simulink model "D53_LKAS_JLU_20200910_1510"  (R2018b)
settings: Solver=ode3  StartTime=0.0  StopTime=10.0  FixedStep=0.01  RelTol=1e-3  EnableMultiTasking=on
model workspace (MAT data in the model file):
  MCOS : class17 (value not decoded)
  MCOS : class17 (value not decoded)
  MCOS : class17 (value not decoded)
  MCOS : class17 (value not decoded)
  MCOS : class17 (value not decoded)
  MCOS : class17 (value not decoded)
  MCOS : class17 (value not decoded)
  MCOS : class17 (value not decoded)
  MCOS : class17 (value not decoded)
  MCOS : class17 (value not decoded)
  MCOS : class17 (value not decoded)
  MCOS : class17 (value not decoded)
  MCOS : class17 (value not decoded)
  MCOS : class17 (value not decoded)
  MCOS : class17 (value not decoded)
  MCOS : class17 (value not decoded)
  MCOS : class17 (value not decoded)
  MCOS : class17 (value not decoded)
  MCOS : class17 (value not decoded)
  MCOS : class17 (value not decoded)
  MCOS : class17 (value not decoded)
  MCOS : class17 (value not decoded)
  MCOS : class17 (value not decoded)
  MCOS : class17 (value not decoded)
  MCOS : class17 (value not decoded)
  MCOS : class17 (value not decoded)
  MCOS : class17 (value not decoded)
  MCOS : class17 (value not decoded)
  MCOS : class17 (value not decoded)
  MCOS : class17 (value not decoded)
  MCOS : class17 (value not decoded)
  MCOS : class17 (value not decoded)
  MCOS : class17 (value not decoded)
  MCOS : class17 (value not decoded)
  MCOS : class17 (value not decoded)
  MCOS : class17 (value not decoded)
  MCOS : class17 (value not decoded)
  MCOS : class17 (value not decoded)
  MCOS : class17 (value not decoded)
  MCOS : class17 (value not decoded)
  MCOS : class17 (value not decoded)
  MCOS : class17 (value not decoded)
  MCOS : class17 (value not decoded)
  MCOS : class17 (value not decoded)
  MCOS : class17 (value not decoded)
  MCOS : class17 (value not decoded)
  MCOS : class17 (value not decoded)
  MCOS : class17 (value not decoded)
  MCOS : class17 (value not decoded)
  MCOS : class17 (value not decoded)
  MCOS : class17 (value not decoded)
  MCOS : class17 (value not decoded)
  MCOS : class17 (value not decoded)
  MCOS : class17 (value not decoded)
  MCOS : class17 (value not decoded)
  MCOS : class17 (value not decoded)
  MCOS : class17 (value not decoded)
  MCOS : class17 (value not decoded)
  MCOS : class17 (value not decoded)
  MCOS : class17 (value not decoded)
  MCOS : class17 (value not decoded)
  MCOS : class17 (value not decoded)
  MCOS : class17 (value not decoded)
  MCOS : class17 (value not decoded)
  MCOS : class17 (value not decoded)
  MCOS : class17 (value not decoded)
  MCOS : class17 (value not decoded)
  MCOS : class17 (value not decoded)
  MCOS : class17 (value not decoded)
  MCOS : class17 (value not decoded)
  MCOS : class17 (value not decoded)
  MCOS : class17 (value not decoded)
  MCOS : class17 (value not decoded)
  MCOS : class17 (value not decoded)
  MCOS : class17 (value not decoded)
  MCOS : class17 (value not decoded)
  MCOS : class17 (value not decoded)
  MCOS : class17 (value not decoded)
  MCOS : class17 (value not decoded)
  MCOS : class17 (value not decoded)
  MCOS : class17 (value not decoded)
  MCOS : class17 (value not decoded)
  MCOS : class17 (value not decoded)
  MCOS : class17 (value not decoded)
  MCOS : class17 (value not decoded)
  MCOS : class17 (value not decoded)
  MCOS : class17 (value not decoded)
  MCOS : class17 (value not decoded)
  MCOS : class17 (value not decoded)
undefined symbols (not defined in the file): LKA_CarWidth, LKA_SampleTime, LKA_StrRatio_C, LKA_Veh2CamL_C, LKA_Veh2CamW_C, LKA_WhlBaseL_C, LL_CompSWA_C, LL_CrvtPrvwT_C, LL_DesDvt_C, LL_DvtComp_C, LL_DvtPrvwT_C, LL_DvtSpdDet_vDvtSpdMin_C, LL_HdAgExT_C, LL_HdAgPrvwT_C, LL_LAccMax_C, LL_LAccRMax_C, LL_LDW_EarliestWarnLine_C, LL_LDW_LatestWarnLine_C, LL_LDWS_SUPPRESS_HEADING, LL_LFClb_TFC_DiffCtlBalance, LL_LFClb_TFC_DiffCtrlMaxSWA, LL_LFClb_TFC_DiffCtrlRatio, LL_LFClb_TFC_facmGainLutGain1_C, LL_LFClb_TFC_facmGainLutGain2_C, LL_LFClb_TFC_facmIntegRatio, LL_LFClb_TFC_facmKlat_C, LL_LFClb_TFC_FfCtlRatio_C, LL_LFClb_TFC_phiIntegCtlMaxSWA_C, LL_LFClb_TFC_tiKlatPrvwT_C, LL_LFClb_TFC_vGainLutVehSpdLwr_C, LL_LFClb_TFC_vGainLutVehSpdUpr_C, LL_LKA_EarliestWarnLine_C, LL_LKA_LatestWarnLine_C, LL_LKAExPrcs_ExitC0Dvt, LL_LKAExPrcs_ExitC0Swt, LL_LKAExPrcs_tiExitTime1, LL_LKAExPrcs_tiExitTime2, LL_LKAExPrcs_tiExitTime3, LL_LKAS_OUT_OF_CONTROL_LAT_VEL, LL_LKAS_OUT_OF_CONTROL_TTLC, LL_LKASWASyn_M0, LL_LKASWASyn_M1, LL_LKASWASyn_M2, LL_LKASWASyn_M3K, LL_LKASWASyn_SWAaddMax, LL_LKASWASyn_T2, LL_LKASWASyn_tiTrqSwaRtTime, LL_LKASWASyn_tiTrqSwaTime, LL_LKASWASyn_TrqMax, LL_LKASWASyn_TrqSwaAddSwt, LL_LKASWASyn_TrqSwaRateDiff, LL_LSpdCompT_C, LL_lStpLngth_C, LL_MAX_DELAY_EPSSTAR_TIME, LL_MAX_DRIVER_TORQUE_DISABLE, LL_MAX_DRIVER_TORQUE_ENABLE, LL_MAX_LANE_WIDTH_DISABLE, LL_MAX_LANE_WIDTH_ENABLE, LL_MAX_LAT_ACC_DISABLE, LL_MAX_LAT_ACC_ENABLE ... (+30)
libraries: simulink x134, canmsglib x52, dspstat3 x3, simulink_extras x1
(part 13 of 18)

== system D53_LKAS_JLU_20200910_1510/LL/LLOn/LL State Determination (LLStateDet)/LL State Machine Conditions (LLSMCon)/Deactivation Condition (DeactvC)/Deactivation Condition Synthesis (DeactvCSyn) ==
  DeactvCSyn_stDACMode : Inport
  DeactvCSyn_stDvtThresActvFlgLDW : Inport  Port=2
  DeactvCSyn_stDvtThresActvFlgLKA : Inport  Port=3
  DvrTkCon_stDvrTkConFlg : Inport  Port=4
  DeactvCSyn_stEPSCFlg : Inport  Port=5
  DeactvCSyn_stExitFlg : Inport  Port=6
  Cast To Single : DataTypeConversion  OutDataTypeStr=uint8
  Cast To Single1 : DataTypeConversion  OutDataTypeStr=uint8
  Default Flag (DflFlg) : Subsystem  TreatAsAtomicUnit=on
  Default Flag (DflFlg)1 : Subsystem  TreatAsAtomicUnit=on
  If : If  NumInputs=2  IfExpression=(u1 ==1|u1==2)& u2 == 0
  If1 : If  NumInputs=4  IfExpression=u1 == 2 & (u3 == 1 | u4 == 1)
  LDW Deactivation Flag (LDWDeactvFlg) : Subsystem  TreatAsAtomicUnit=on
  LKA Deactivation Flag (LKADeactvFlg) : Subsystem  TreatAsAtomicUnit=on
  Logical Operator : Logic  Operator=OR  AllPortsSameDT=off  OutDataTypeStr=boolean
  Merge : Merge
  Merge1 : Merge
  DeactvCSyn_stLDWDeactvCSyn : Outport
  DeactvCSyn_stLKADeactvCSyn : Outport  Port=2
  wires:
  DeactvCSyn_stDvtThresActvFlgLDW/1 -> If/2
  Logical Operator/1 -> Cast To Single/1
  DvrTkCon_stDvrTkConFlg/1 -> Logical Operator/1
  Cast To Single/1 -> If1/3
  If1/1 -> LKA Deactivation Flag (LKADeactvFlg)/Action
  Default Flag (DflFlg)1/1(Out) -> Merge1/2
  LKA Deactivation Flag (LKADeactvFlg)/1(Out) -> Merge1/1
  DeactvCSyn_stExitFlg/1 -> Cast To Single1/1
  DeactvCSyn_stEPSCFlg/1 -> Logical Operator/2
  Merge1/1 -> DeactvCSyn_stLKADeactvCSyn/1
  If1/2 -> Default Flag (DflFlg)1/Action
  Default Flag (DflFlg)/1(Out) -> Merge/2
  Merge/1 -> DeactvCSyn_stLDWDeactvCSyn/1
  DeactvCSyn_stDvtThresActvFlgLKA/1 -> If1/2
  DeactvCSyn_stDACMode/1 -> If/1, If1/1
  If/2 -> Default Flag (DflFlg)/Action
  If/1 -> LDW Deactivation Flag (LDWDeactvFlg)/Action
  LDW Deactivation Flag (LDWDeactvFlg)/1(Out) -> Merge/1
  Cast To Single1/1 -> If1/4

== system D53_LKAS_JLU_20200910_1510/LL/LLOn/LL State Determination (LLStateDet)/LL State Machine Conditions (LLSMCon)/Deactivation Condition (DeactvC)/Deviation Threshold Condition (DvtThresCon) ==
  DvtThresCon_vVehSpd : Inport
  DvtThresCon_bsL0Info : Inport  Port=2
  DvtThresCon_bsR0Info : Inport  Port=3
  DvtThresCon_bsTTLCInfo : Inport  Port=4
  DvtThresCon_bsHdAgInfo : Inport  Port=5
  DvtThresCon_bsDvtThresClb : Inport  Port=6
  Active Lane Calculation (ActLanCalc) : Subsystem
  Bus Selector : BusSelector  OutputSignals=LftTTLC,RgtTTLC
  Bus Selector1 : BusSelector  OutputSignals=ActvCClb
  Bus Selector2 : BusSelector  OutputSignals=phiHdAgLft,phiHdAgRgt
  Deviation Calculation (DvtCalc) : Subsystem
  Deviation Speed Calculation (DvtSpdCalc) : Subsystem
  Deviation Threshold Judgement LDW (DvtThresJdg) : Subsystem
  Deviation Threshold Judgement LKA (DvtThresJdg) : Subsystem
  Saturation1 : Saturate  UpperLimit=1  LowerLimit=-1
  Saturation5 : Saturate  UpperLimit=1  LowerLimit=-1
  DvtThresCon_stDvtThresActvFlgLDW : Outport
  DvtThresCon_stDvtThresActvFlgLKA : Outport  Port=2
  wires:
  Saturation1/1 -> Deviation Threshold Judgement LDW (DvtThresJdg)/2(DvtThresJdg_lRgtDvt), Deviation Threshold Judgement LKA (DvtThresJdg)/2(DvtThresJdg_lRgtDvt)
  Bus Selector/1 -> Deviation Threshold Judgement LDW (DvtThresJdg)/5(DvtThresJdg_tiLftTTLC), Deviation Threshold Judgement LKA (DvtThresJdg)/5(DvtThresJdg_tiLftTTLC)  "<LftTTLC>"
  Saturation5/1 -> Deviation Threshold Judgement LDW (DvtThresJdg)/1(DvtThresJdg_lLftDvt), Deviation Threshold Judgement LKA (DvtThresJdg)/1(DvtThresJdg_lLftDvt)
  Deviation Speed Calculation (DvtSpdCalc)/2(DvtSpdCalc_vRgtDvtSpd) -> Deviation Threshold Judgement LDW (DvtThresJdg)/4(DvtThresJdg_vRgtDvtSpd), Deviation Threshold Judgement LKA (DvtThresJdg)/4(DvtThresJdg_vRgtDvtSpd)  "DvtSpdCalc_vRgtDvtSpd"
  Bus Selector/2 -> Deviation Threshold Judgement LDW (DvtThresJdg)/6(DvtThresJdg_tiRgtTTLC), Deviation Threshold Judgement LKA (DvtThresJdg)/6(DvtThresJdg_tiRgtTTLC)  "<RgtTTLC>"
  Deviation Speed Calculation (DvtSpdCalc)/1(DvtSpdCalc_vLftDvtSpd) -> Deviation Threshold Judgement LDW (DvtThresJdg)/3(DvtThresJdg_vLftDvtSpd), Deviation Threshold Judgement LKA (DvtThresJdg)/3(DvtThresJdg_vLftDvtSpd)  "DvtSpdCalc_vLftDvtSpd"
  Active Lane Calculation (ActLanCalc)/1(ActLanCalc_ActvCClbOut) -> Deviation Threshold Judgement LDW (DvtThresJdg)/7(DvtThresJdg_bsDvtThresClb), Deviation Threshold Judgement LKA (DvtThresJdg)/7(DvtThresJdg_bsDvtThresClb)
  Deviation Threshold Judgement LDW (DvtThresJdg)/1(DvtThresJdg_stDvtThresActvFlg) -> DvtThresCon_stDvtThresActvFlgLDW/1  "DvtThresActvFlg"
  Bus Selector2/2 -> Deviation Speed Calculation (DvtSpdCalc)/2(DvtSpdCalc_phiPrvwHdAgRgt)  "<phiHdAgRgt>"
  Bus Selector2/1 -> Deviation Speed Calculation (DvtSpdCalc)/1(DvtSpdCalc_phiPrvwHdAgLft)  "<phiHdAgLft>"
  DvtThresCon_bsHdAgInfo/1 -> Bus Selector2/1
  DvtThresCon_bsTTLCInfo/1 -> Bus Selector/1  "TTLCInfo"
  DvtThresCon_vVehSpd/1 -> Deviation Speed Calculation (DvtSpdCalc)/3(DvtSpdCalc_vVehSpd)
  DvtThresCon_bsDvtThresClb/1 -> Bus Selector1/1
  Deviation Threshold Judgement LKA (DvtThresJdg)/1(DvtThresJdg_stDvtThresActvFlg) -> DvtThresCon_stDvtThresActvFlgLKA/1  "DvtThresActvFlg"
  Deviation Calculation (DvtCalc)/2(DvtCalc_lRgtDvt) -> Saturation1/1  "DvtCalc_lRgtDvt"
  Deviation Calculation (DvtCalc)/1(DvtCalc_lLftDvt) -> Saturation5/1  "DvtCalc_lLftDvt"
  DvtThresCon_bsR0Info/1 -> Active Lane Calculation (ActLanCalc)/2(ActLanCalc_bsR0Info), Deviation Calculation (DvtCalc)/2(DvtCalc_bsR0Info)
  DvtThresCon_bsL0Info/1 -> Active Lane Calculation (ActLanCalc)/1(ActLanCalc_bsL0Info), Deviation Calculation (DvtCalc)/1(DvtCalc_bsL0Info)
  Bus Selector1/1 -> Active Lane Calculation (ActLanCalc)/3(ActLanCalc_ActvCClb)  "<ActvCClb>"

== system D53_LKAS_JLU_20200910_1510/LL/LLOn/LL State Determination (LLStateDet)/LL State Machine Conditions (LLSMCon)/Deactivation Condition (DeactvC)/Driver Take Condition (DvrTkCon) ==
  DvrTkCon_crPrvwCrvt : Inport
  DvrTkCon_stActvFlg : Inport  Port=2
  DvrTkCon_bsLLSMConClb : Inport  Port=3
  DvrTkCon_vVehSpd : Inport  Port=4
  DvrTkCon_bsEPSInfo : Inport  Port=5
  Abs1 : Abs
  Add : Sum
  Bus Selector1 : BusSelector  OutputSignals=EPS_SW_Trq
  Bus Selector2 : BusSelector  OutputSignals=DisblCClb.LL_MAX_DRIVER_TORQUE_DISABLE
  Bus Selector3 : BusSelector  OutputSignals=LKA_SampleTime
  Cast To Single : DataTypeConversion  OutDataTypeStr=uint16
  Cast To Single1 : DataTypeConversion  OutDataTypeStr=uint16
  Cast To Single2 : DataTypeConversion  LockScale=on
  Compare To Constant : simulink/Logic and Bit Operations/Compare To Constant  relop=>  const=0  OutDataTypeStr=boolean
  Constant : Constant  Value=0.005  OutDataTypeStr=single
  Constant1 : Constant  OutDataTypeStr=single
  Constant2 : Constant  Value=0.2  OutDataTypeStr=single
  Count : Subsystem
  Count 0.2s : Subsystem
  Divide : Product  Inputs=*/
  Divide1 : Product  Inputs=*/
  Divide2 : Product  Inputs=*/  OutDataTypeStr=single
  Logical Operator : Logic  AllPortsSameDT=off  OutDataTypeStr=boolean
  MATLAB Function : MATLAB Function  TreatAsAtomicUnit=on
  Memory : Memory  InheritSampleTime=on
  Saturation : Saturate  UpperLimit=0.005  LowerLimit=-0.005
  Time Delay (TDel) : Subsystem
  DvrTkCon_stDvrTkConFlg : Outport
  wires:
  Count/1(Out) -> Add/2
  Cast To Single1/1 -> Add/1
  Memory/1 -> Logical Operator/2
  Logical Operator/1 -> Count/Enable
  Compare To Constant/1 -> Count/1(Input), Logical Operator/1
  Add/1 -> Time Delay (TDel)/2(TDel_tiTDel)
  Cast To Single/1 -> Count 0.2s/2(Input1)
  Bus Selector2/1 -> MATLAB Function/4(DisableTrq)  "<LL_MAX_DRIVER_TORQUE_DISABLE>"
  Saturation/1 -> Abs1/1
  DvrTkCon_crPrvwCrvt/1 -> Saturation/1
  Divide2/1 -> Cast To Single2/1
  Constant/1 -> Divide2/2
  Cast To Single2/1 -> MATLAB Function/5(CrvtTrq)
  Abs1/1 -> Divide2/1
  Divide1/1 -> Cast To Single1/1
  Constant1/1 -> Divide1/1
  Constant2/1 -> Divide/1
  Bus Selector3/1 -> Divide/2, Divide1/2  "<LKA_SampleTime>"
  Divide/1 -> Cast To Single/1
  [LLClb_bsConstantClb] -> Bus Selector3/1
  Time Delay (TDel)/1(TDel_stFlgOut) -> Memory/1, DvrTkCon_stDvrTkConFlg/1
  Count 0.2s/1(Out) -> Time Delay (TDel)/1(TDel_stFlgIn)
  MATLAB Function/1(stDvrTkConFlg) -> Count 0.2s/1(Input), Count 0.2s/Enable
  DvrTkCon_bsLLSMConClb/1 -> Bus Selector2/1
  DvrTkCon_vVehSpd/1 -> MATLAB Function/3(VehSpd)
  Bus Selector1/1 -> MATLAB Function/2(EPSTrq)  "<EPS_SW_Trq>"
  DvrTkCon_stActvFlg/1 -> MATLAB Function/1(stActvFlg), Compare To Constant/1
  DvrTkCon_bsEPSInfo/1 -> Bus Selector1/1

== system D53_LKAS_JLU_20200910_1510/LL/LLOn/LL State Determination (LLStateDet)/LL State Machine Conditions (LLSMCon)/Deactivation Condition (DeactvC)/EPS Condition (EPSC) ==
  EPSC_bsLLSMConClb : Inport
  EPSC_bsEPSInfo : Inport  Port=2
  EPSC_bsLLState : Inport  Port=3
  Bus Selector : BusSelector  OutputSignals=EPS_LKA_State
  Bus Selector1 : BusSelector  OutputSignals=LKA_State
  Bus Selector2 : BusSelector  OutputSignals=DisblCClb.LL_TkOvStChk_tiTDelTime
  Bus Selector3 : BusSelector  OutputSignals=LKA_SampleTime
  Cast To Single1 : DataTypeConversion  OutDataTypeStr=uint16
  Compare To Constant : simulink/Logic and Bit Operations/Compare To Constant  relop=~=  const=3  OutDataTypeStr=boolean
  Compare To Constant1 : simulink/Logic and Bit Operations/Compare To Constant  relop===  const=4  OutDataTypeStr=boolean
  Compare To Constant2 : simulink/Logic and Bit Operations/Compare To Constant  relop===  const=5  OutDataTypeStr=boolean
  Divide : Product  Inputs=*/  OutDataTypeStr=single
  Logical Operator : Logic  Operator=OR  AllPortsSameDT=off  OutDataTypeStr=boolean
  Logical Operator1 : Logic  AllPortsSameDT=off  OutDataTypeStr=boolean
  Sum Condition1 : Subsystem  TreatAsAtomicUnit=on
  EPSC_stEPSCFlg : Outport
  wires:
  Cast To Single1/1 -> Sum Condition1/2(Sum)
  EPSC_bsLLSMConClb/1 -> Bus Selector2/1
  Divide/1 -> Cast To Single1/1
  [LLClb_bsConstantClb] -> Bus Selector3/1
  Bus Selector2/1 -> Divide/1  "<LL_TkOvStChk_tiTDelTime>"
  Bus Selector3/1 -> Divide/2  "<LKA_SampleTime>"
  Sum Condition1/1(Out) -> Logical Operator1/2
  Logical Operator/1 -> Sum Condition1/Enable, Sum Condition1/1(In)
  Compare To Constant/1 -> Logical Operator1/1
  Compare To Constant2/1 -> Logical Operator/2
  Compare To Constant1/1 -> Logical Operator/1
  Bus Selector1/1 -> Compare To Constant2/1, Compare To Constant1/1  "<LKA_State>"
  Bus Selector/1 -> Compare To Constant/1  "<EPS_LKA_State>"
  EPSC_bsLLState/1 -> Bus Selector1/1
  Logical Operator1/1 -> EPSC_stEPSCFlg/1
  EPSC_bsEPSInfo/1 -> Bus Selector/1

== system D53_LKAS_JLU_20200910_1510/LL/LLOn/LL State Determination (LLStateDet)/LL State Machine Conditions (LLSMCon)/Disable Condition (DisblC)/Disable Condition Synthesis (DisblCSyn) ==
  DisblCSyn_stDACMode : Inport
  DisblCSyn_stVehStateC : Inport  Port=2
  DisblCSyn_stLaneC : Inport  Port=3
  DisblCSyn_stDrvInttC : Inport  Port=4
  DisblCSyn_stLDWOwnC : Inport  Port=5
  DisblCSyn_stLKAOwnC : Inport  Port=6
  DisblCSyn_stLDWAlrmTOut : Inport  Port=7
  Cast To Single : DataTypeConversion  OutDataTypeStr=uint8
  Cast To Single1 : DataTypeConversion  OutDataTypeStr=uint8
  Cast To Single2 : DataTypeConversion  OutDataTypeStr=uint8
  If Action Subsystem1 : Subsystem  TreatAsAtomicUnit=on
  If Action Subsystem2 : Subsystem  TreatAsAtomicUnit=on
  If Action Subsystem3 : Subsystem  TreatAsAtomicUnit=on
  If Action Subsystem4 : Subsystem  TreatAsAtomicUnit=on
  If1 : If  NumInputs=2  IfExpression=(u1 ==1|u1==2)& u2 == 1
  If2 : If  NumInputs=2  IfExpression=u1 == 2 & u2 == 1
  Logical Operator1 : Logic  Operator=OR  AllPortsSameDT=off  OutDataTypeStr=boolean
  Logical Operator2 : Logic  Operator=OR  Inputs=3  AllPortsSameDT=off  OutDataTypeStr=boolean
  Logical Operator3 : Logic  Operator=OR  Inputs=3  AllPortsSameDT=off  OutDataTypeStr=boolean
  Merge1 : Merge
  Merge2 : Merge
  DisblCSyn_stLDWDisblCSyn : Outport
  DisblCSyn_stLKADisblCSyn : Outport  Port=2
  wires:
  Cast To Single2/1 -> If2/2
  Cast To Single1/1 -> If1/2
  Cast To Single/1 -> If1/1, If2/1
  DisblCSyn_stLDWAlrmTOut/1 -> Logical Operator3/2
  Merge2/1 -> DisblCSyn_stLKADisblCSyn/1
  Logical Operator1/1 -> Cast To Single2/1
  If Action Subsystem3/1(Out) -> Merge2/2
  If2/2 -> If Action Subsystem3/Action
  If2/1 -> If Action Subsystem1/Action
  If Action Subsystem1/1(Out) -> Merge2/1
  DisblCSyn_stLKAOwnC/1 -> Logical Operator1/2
  If Action Subsystem4/1(Out) -> Merge1/2
  Merge1/1 -> DisblCSyn_stLDWDisblCSyn/1
  If1/2 -> If Action Subsystem4/Action
  If1/1 -> If Action Subsystem2/Action
  If Action Subsystem2/1(Out) -> Merge1/1
  Logical Operator2/1 -> Logical Operator1/1, Logical Operator3/3
  DisblCSyn_stDACMode/1 -> Cast To Single/1
  Logical Operator3/1 -> Cast To Single1/1
  DisblCSyn_stLDWOwnC/1 -> Logical Operator3/1
  DisblCSyn_stDrvInttC/1 -> Logical Operator2/3
  DisblCSyn_stLaneC/1 -> Logical Operator2/2
  DisblCSyn_stVehStateC/1 -> Logical Operator2/1

== system D53_LKAS_JLU_20200910_1510/LL/LLOn/LL State Determination (LLStateDet)/LL State Machine Conditions (LLSMCon)/Disable Condition (DisblC)/Driver Intent Condition (DrvInttC) ==
  DrvInttC_bsInInfoSyn : Inport
  DrvInttC_bsLLSMConClb : Inport  Port=2
  DrvInttC_crPrvwCrvt : Inport  Port=3
  Bus Creator : BusCreator  Inputs=3
  Bus Selector : BusSelector  OutputSignals=bsSWAInfo.SW_Angle,bsVehMovInfo.ESC_LatAcc,bsVehMovInfo.ESC_LonAcc,bsEPSInfo,bsVehMovInfo.ESC_VehSpd
  Bus Selector1 : BusSelector  OutputSignals=DisblCClb.LL_MAX_STEER_ANGLE_DISABLE,DisblCClb.LL_MAX_STEER_SPEED_DISABLE,DisblCClb.LL_MAX_DRIVER_TORQUE_DISABLE,DisblCClb.LL_MAX_LAT_ACC_DISABLE,DisblCClb.LL_MAX_LONG_ACC_DISABLE,DisblCClb.LL_MAX_LONG_DECEL_DISABLE,DisblCClb.LL_TkOvStChk_tiTrqChkT,DisblCClb.LL_TkOvStChk_tiTDelTime
  Driver Action Condition Synthesis (DrvActnCSyn) : Subsystem  Description=|
      | Block Name: Driver Action Condition Synthesis
      | Ab.: DrvActnCSyn
      | No.: 1.1.1.3.3.5
      | Rev: 0.0.1
      | Update Date: 19-3-26
  Driver Action Detection (DrvActnDet) : Subsystem  Description=|
      | Block Name: Driver Action Detection
      | Ab.: DrvActnDet
      | No.: 1.1.1.3.3.1
      | Rev: 0.0.1
      | Update Date: 19-3-26
  Driver Release Detection (DrvRlsDet) : Subsystem  Description=|
      | Block Name: Driver Release Detection
      | Ab.: DrvRlsDet
      | No.: 1.1.1.2.3.2
      | Rev: 0.0.1
      | Update Date: 19-3-26
  Take-Over Steering Check (TkOvStChk) : Subsystem  Description=|
      | Block Name: Take-Over Steering Check
      | Ab.: TkOvStChk
      | No.: 1.1.1.3.3.4
      | Rev: 0.0.1
      | Update Date: 19-3-26
  DrvInttC_stDrvInttCSyn : Outport
  DrvInttCSyn : Outport  Port=2
  wires:
  Bus Creator/1 -> DrvInttCSyn/1
  Driver Action Detection (DrvActnDet)/2(DrvActnDet) -> Bus Creator/1  "DrvActnDet"
  Driver Release Detection (DrvRlsDet)/1(DrvRlsDet_stDrvRlsDetFlg) -> Driver Action Condition Synthesis (DrvActnCSyn)/2(DrvActnCSyn_stDrvRlsDetFlg), Bus Creator/2  "DRIVER_RELEASE"
  Take-Over Steering Check (TkOvStChk)/1(TkOvStChk_stTkOvStChk) -> Driver Action Condition Synthesis (DrvActnCSyn)/3(DrvActnCSyn_stTkOvStChk), Bus Creator/3  "TkOvStChk"
  DrvInttC_crPrvwCrvt/1 -> Take-Over Steering Check (TkOvStChk)/6(TkOvStChk_crPrvwCrvt)
  DrvInttC_bsInInfoSyn/1 -> Bus Selector/1
  Bus Selector/5 -> Take-Over Steering Check (TkOvStChk)/1(TkOvStChk_bsVehSpd)  "<ESC_VehSpd>"
  Bus Selector1/8 -> Take-Over Steering Check (TkOvStChk)/5(TkOvStChk_tiTDel_C)  "<LL_TkOvStChk_tiTDelTime>"
  Bus Selector1/7 -> Take-Over Steering Check (TkOvStChk)/4(TkOvStChk_tiTrqChkT_C)  "<LL_TkOvStChk_tiTrqChkT>"
  Bus Selector1/3 -> Take-Over Steering Check (TkOvStChk)/3(TkOvStChk_trqSWTrqMax_C)  "<LL_MAX_DRIVER_TORQUE_DISABLE>"
  Bus Selector/4 -> Driver Action Detection (DrvActnDet)/9(DrvActnDet_bsEPSInfo), Driver Release Detection (DrvRlsDet)/1(DrvRlsDet_bsEPSInfo), Take-Over Steering Check (TkOvStChk)/2(TkOvStChk_bsEPSInfo)  "<bsEPSInfo>"
  Bus Selector1/6 -> Driver Action Detection (DrvActnDet)/8(DrvActnDet_aFAccMin_C)  "<LL_MAX_LONG_DECEL_DISABLE>"
  Bus Selector1/5 -> Driver Action Detection (DrvActnDet)/7(DrvActnDet_aFAccMax_C)  "<LL_MAX_LONG_ACC_DISABLE>"
  Bus Selector1/4 -> Driver Action Detection (DrvActnDet)/6(DrvActnDet_aLAccMax_C)  "<LL_MAX_LAT_ACC_DISABLE>"
  Bus Selector1/2 -> Driver Action Detection (DrvActnDet)/5(DrvActnDet_dphiSWARateMax_C)  "<LL_MAX_STEER_SPEED_DISABLE>"
  Bus Selector1/1 -> Driver Action Detection (DrvActnDet)/4(DrvActnDet_phiSWAMax_C)  "<LL_MAX_STEER_ANGLE_DISABLE>"
  DrvInttC_bsLLSMConClb/1 -> Bus Selector1/1
  Bus Selector/3 -> Driver Action Detection (DrvActnDet)/3(DrvActnDet_aFAcc)  "<ESC_LonAcc>"
  Bus Selector/2 -> Driver Action Detection (DrvActnDet)/2(DrvActnDet_aLAcc)  "<ESC_LatAcc>"
  Bus Selector/1 -> Driver Action Detection (DrvActnDet)/1(DrvActnDet_phiSWA)  "<SW_Angle>"
  Driver Action Detection (DrvActnDet)/1(DrvActnDet_stTkOvStActvFlg) -> Driver Action Condition Synthesis (DrvActnCSyn)/1(DrvActnCSyn_stTkOvStActvFlg)  "DRIVER_ACT"
  Driver Action Condition Synthesis (DrvActnCSyn)/1(DrvActnCSyn_stDrvActnCSyn) -> DrvInttC_stDrvInttCSyn/1  "DRIVER"

== system D53_LKAS_JLU_20200910_1510/LL/LLOn/LL State Determination (LLStateDet)/LL State Machine Conditions (LLSMCon)/Disable Condition (DisblC)/LDW Alarm Timeout (LDWAlrmTOut) ==
  LDWAlrmTOut_bsLLState : Inport
  LDWAlrmTOut_bsLLSMConClb : Inport  Port=2
  Bus Selector : BusSelector  OutputSignals=LDW_State
  Bus Selector1 : BusSelector  OutputSignals=DisblCClb.LL_Max_LDWS_Warning_Time
  Bus Selector2 : BusSelector  OutputSignals=LKA_SampleTime
  Cast To Single1 : DataTypeConversion  OutDataTypeStr=uint16
  Divide : Product  Inputs=*/
  If Action Subsystem : Subsystem  TreatAsAtomicUnit=on
  If Action Subsystem1 : Subsystem  TreatAsAtomicUnit=on
  Memory : Memory  InheritSampleTime=on
  Merge : Merge
  u1>=3|u1==1&u2==u3 : If  NumInputs=3  IfExpression=u1==4|u1==5&u2==u3
  LDWAlrmTOut_stLDWAlrmTOut : Outport
  wires:
  Cast To Single1/1 -> If Action Subsystem/1(In)
  [LLClb_bsConstantClb] -> Bus Selector2/1
  Bus Selector2/1 -> Divide/2  "<LKA_SampleTime>"
  Merge/1 -> LDWAlrmTOut_stLDWAlrmTOut/1
  Divide/1 -> Cast To Single1/1
  Bus Selector1/1 -> Divide/1  "<LL_Max_LDWS_Warning_Time>"
  LDWAlrmTOut_bsLLSMConClb/1 -> Bus Selector1/1
  Bus Selector/1 -> Memory/1, u1>=3|u1==1&u2==u3/3, u1>=3|u1==1&u2==u3/1  "<LDW_State>"
  LDWAlrmTOut_bsLLState/1 -> Bus Selector/1
  If Action Subsystem/1(Out) -> Merge/1
  u1>=3|u1==1&u2==u3/2 -> If Action Subsystem1/Action
  u1>=3|u1==1&u2==u3/1 -> If Action Subsystem/Action
  If Action Subsystem1/1(Out1) -> Merge/2
  Memory/1 -> u1>=3|u1==1&u2==u3/2

== system D53_LKAS_JLU_20200910_1510/LL/LLOn/LL State Determination (LLStateDet)/LL State Machine Conditions (LLSMCon)/Disable Condition (DisblC)/LDW Own Condition (LDWOwnC) ==
  LDWOwnC_stDACMode : Inport
  LDWOwnC_bsPrDvtInfo : Inport  Port=2
  LDWOwnC_bsLLSMConClb : Inport  Port=3
  Bus Selector1 : BusSelector  OutputSignals=EnaCClb.LL_LDW_LatestWarnLine_C
  LDW Own Condition Synthesis (LDWOwnCSyn) : Subsystem  Description=|
      | Block Name: LDW Own Condition Synthesis
      | Ab.: LDWOwnCSyn
      | No.: 1.1.1.3.4.2
      | Rev: 0.0.1
      | Update Date: 19-3-26
  Vehicle Position Check (VehPosChk) : Subsystem  Description=|
      | Block Name: Vehicle Position Check
      | Ab.: VehPosChk
      | No.: 1.1.1.3.4.1
      | Rev: 0.0.1
      | Update Date: 19-3-26
  LDWOwnC_stLDWOwnCSyn : Outport
  wires:
  LDWOwnC_bsPrDvtInfo/1 -> Vehicle Position Check (VehPosChk)/1(VehPosChk_bsPrDvtInfo)
  Bus Selector1/1 -> Vehicle Position Check (VehPosChk)/2(VehPosChk_LatestLine_C)  "<LL_LDW_LatestWarnLine_C>"
  LDWOwnC_bsLLSMConClb/1 -> Bus Selector1/1
  LDWOwnC_stDACMode/1 -> LDW Own Condition Synthesis (LDWOwnCSyn)/1(LDWOwnCSyn_stDACMode)
  Vehicle Position Check (VehPosChk)/1(VehPosChk_stVehPosChk) -> LDW Own Condition Synthesis (LDWOwnCSyn)/2(LDWOwnCSyn_stVehPosChk)
  LDW Own Condition Synthesis (LDWOwnCSyn)/1(LDWOwnCSyn_stLDWOwnCSyn) -> LDWOwnC_stLDWOwnCSyn/1

== system D53_LKAS_JLU_20200910_1510/LL/LLOn/LL State Determination (LLStateDet)/LL State Machine Conditions (LLSMCon)/Disable Condition (DisblC)/LKA Own Condition (LKAOwnC) ==
  LKAOwnC_stDACMode : Inport
  LKAOwnC_bsInInfoSyn : Inport  Port=2
  LKAOwnC_bsTTLCInfo : Inport  Port=3
  LKAOwnC_bsLLState : Inport  Port=4
  LKAOwnC_bsLLSMConClb : Inport  Port=5
  Bus Creator : BusCreator  Inputs=3
  Bus Selector : BusSelector  OutputSignals=bsLaneInfo.bsL0Info,bsLaneInfo.bsR0Info,bsEPSInfo
  Bus Selector1 : BusSelector  OutputSignals=EnaCClb.LL_LKAS_OUT_OF_CONTROL_LAT_VEL,EnaCClb.LL_DvtComp_C,EnaCClb.LL_LKA_LatestWarnLine_C,DisblCClb.LL_MAX_DELAY_EPSSTAR_TIME
  EPS Condition (EPSC) : Subsystem  Description=|
      | Block Name: EPS Condition
      | Ab.: EPSC
      | No.: 1.1.1.3.5.3
      | Rev: 0.0.1
      | Update Date: 19-3-26
  LKA Own Condition Synthesis (LKAOwnCSyn) : Subsystem  Description=|
      | Block Name: LKA Own Condition Synthesis
      | Ab.: LKAOwnCSyn
      | No.: 1.1.1.3.5.4
      | Rev: 0.0.1
      | Update Date: 19-3-26
  Vehicle Lateral Speed Condition (VehLSpdC) : Subsystem  Description=|
      | Block Name: Vehicle Lateral Speed Condition
      | Ab.: VehLSpdC
      | No.: 1.1.1.3.5.1
      | Rev: 0.0.1
      | Update Date: 19-3-26
  Vehicle Position Check (VehPosChk) : Subsystem  Description=|
      | Block Name: Vehicle Position Check
      | Ab.: VehPosChk
      | No.: 1.1.1.3.5.2
      | Rev: 0.0.1
      | Update Date: 19-3-26
  LKAOwnC_stLKAOwnCSyn : Outport
  LKAOwnC : Outport  Port=2
  wires:
  Vehicle Lateral Speed Condition (VehLSpdC)/1(VehLSpdC_stVehLSpdC) -> LKA Own Condition Synthesis (LKAOwnCSyn)/2(LKAOwnCSyn_stVehLSpdC), Bus Creator/1  "LKAOWN_VEHLATSPEED"
  EPS Condition (EPSC)/1(EPSC_stEPSC) -> Bus Creator/3, LKA Own Condition Synthesis (LKAOwnCSyn)/4(LKAOwnCSyn_stEPSCtlEC)  "LKAOWN_EPS"
  Vehicle Position Check (VehPosChk)/1(VehPosChk_stVehPosChk) -> LKA Own Condition Synthesis (LKAOwnCSyn)/3(LKAOwnCSyn_stVehPosChk), Bus Creator/2  "LKAOWN_VEHPOS"
  Bus Creator/1 -> LKAOwnC/1
  LKAOwnC_bsTTLCInfo/1 -> Vehicle Lateral Speed Condition (VehLSpdC)/1(VehLSpdC_bsTTLC)
  LKA Own Condition Synthesis (LKAOwnCSyn)/1(LKAOwnCSyn_stLKAOwnCSyn) -> LKAOwnC_stLKAOwnCSyn/1  "LKAOWN"
  Bus Selector1/4 -> EPS Condition (EPSC)/3(EPSC_tiDelT_C)  "<LL_MAX_DELAY_EPSSTAR_TIME>"
  Bus Selector1/3 -> Vehicle Position Check (VehPosChk)/4(VehPosChk_lAlrmLine_C)  "<LL_LKA_LatestWarnLine_C>"
  Bus Selector1/2 -> Vehicle Position Check (VehPosChk)/3(VehPosChk_DvtComp_C)  "<LL_DvtComp_C>"
  Bus Selector1/1 -> Vehicle Lateral Speed Condition (VehLSpdC)/2(VehLSpdC_vVehLSpdMax_C)  "<LL_LKAS_OUT_OF_CONTROL_LAT_VEL>"
  LKAOwnC_bsLLSMConClb/1 -> Bus Selector1/1
  Bus Selector/3 -> EPS Condition (EPSC)/1(EPSC_bsEPSInfo)  "<bsEPSInfo>"
  Bus Selector/2 -> Vehicle Position Check (VehPosChk)/2(VehPosChk_bsR0Info)  "<bsR0Info>"
  Bus Selector/1 -> Vehicle Position Check (VehPosChk)/1(VehPosChk_bsL0Info)  "<bsL0Info>"
  LKAOwnC_stDACMode/1 -> LKA Own Condition Synthesis (LKAOwnCSyn)/1(LKAOwnCSyn_stDACMode)
  LKAOwnC_bsLLState/1 -> EPS Condition (EPSC)/2(EPSC_bsLLState)
  LKAOwnC_bsInInfoSyn/1 -> Bus Selector/1

== system D53_LKAS_JLU_20200910_1510/LL/LLOn/LL State Determination (LLStateDet)/LL State Machine Conditions (LLSMCon)/Disable Condition (DisblC)/Lane Condition (LaneC) ==
  LaneC_bsInInfoSyn : Inport
  LaneC_LaneWidth : Inport  Port=2
  LaneC_crPrvwCrvt : Inport  Port=3
  LaneC_bsLLSMConClb : Inport  Port=4
  Bus Creator : BusCreator  Inputs=4
  Bus Selector : BusSelector  OutputSignals=bsLaneInfo.bsL0Info.L0_Q,bsLaneInfo.bsR0Info.R0_Q,bsLaneInfo.bsL0Info.L0_C1,bsLaneInfo.bsR0Info.R0_C1
  Bus Selector1 : BusSelector  OutputSignals=DisblCClb.LL_MAX_LANE_WIDTH_DISABLE,DisblCClb.LL_MIN_LANE_WIDTH_DISABLE,DisblCClb.LL_MAX_SYSTEM_CURVATURE_DISABLE
  Lane C1 Detection (LaneC1Det) : Subsystem  Description=|
      | Block Name: Lane Width Detection
      | Ab.: LaneWDet
      | No.: 1.1.1.3.2.2
      | Rev: 0.0.1
      | Update Date: 19-3-26
  Lane Condition Synthesis (LaneCSyn) : Subsystem  Description=|
      | Block Name: Lane Condition Synthesis
      | Ab.: LaneCSyn
      | No.: 1.1.1.3.2.4
      | Rev: 0.0.1
      | Update Date: 19-3-26
  Lane Curvature Detection (LaneCrvtDet) : Subsystem  Description=|
      | Block Name: Lane Curvature Detection
      | Ab.: LaneCrvtDet
      | No.: 1.1.1.3.2.3
      | Rev: 0.0.1
      | Update Date: 19-3-26
  Lane Quality Disable Condition (LaneQlDC) : Subsystem  Description=|
      | Block Name: Lane Quality Disable Condition
      | Ab.: LaneQlDC
      | No.: 1.1.1.3.2.1
      | Rev: 0.0.1
      | Update Date: 19-3-26
  Lane Width Detection (LaneWDet) : Subsystem  Description=|
      | Block Name: Lane Width Detection
      | Ab.: LaneWDet
      | No.: 1.1.1.3.2.2
      | Rev: 0.0.1
      | Update Date: 19-3-26
  LaneC_stLanCSyn : Outport
  LanCSyn : Outport  Port=2
  wires:
  Lane Curvature Detection (LaneCrvtDet)/1(LaneCrvtDet_stLaneCrvtDetFlg) -> Bus Creator/3, Lane Condition Synthesis (LaneCSyn)/3(LaneCSyn_stLaneCrvtDetFlg)  "LANE_CURVAT"
  Bus Creator/1 -> LanCSyn/1
  Lane Quality Disable Condition (LaneQlDC)/1(LaneQlDC_stLaneQlDCFlg) -> Lane Condition Synthesis (LaneCSyn)/1(LaneCSyn_stLaneQlECFlg), Bus Creator/1  "LANE_Q"
  Lane C1 Detection (LaneC1Det)/1(LaneC1Det_stLaneC1DetFlg) -> Lane Condition Synthesis (LaneCSyn)/4(LaneCSyn_stLaneC1DetFlg), Bus Creator/4  "LANE_C1"
  LaneC_LaneWidth/1 -> Lane Width Detection (LaneWDet)/1(LaneWDet_LaneWidth)
  Bus Selector/4 -> Lane C1 Detection (LaneC1Det)/2(LaneWDet_facmR0C1)  "<R0_C1>"
  Bus Selector/3 -> Lane C1 Detection (LaneC1Det)/1(LaneWDet_facmL0C1)  "<L0_C1>"
  LaneC_crPrvwCrvt/1 -> Lane Curvature Detection (LaneCrvtDet)/1(LaneCrvtDet_crPrvwCrvt)
  Bus Selector1/3 -> Lane Curvature Detection (LaneCrvtDet)/2(LaneCrvtDet_crLaneCrvtMax_C)  "<LL_MAX_SYSTEM_CURVATURE_DISABLE>"
  LaneC_bsLLSMConClb/1 -> Bus Selector1/1
  Bus Selector1/2 -> Lane Width Detection (LaneWDet)/3(LaneWDet_lLaneWMin)  "<LL_MIN_LANE_WIDTH_DISABLE>"
  Bus Selector1/1 -> Lane Width Detection (LaneWDet)/2(LaneWDet_lLaneWMax)  "<LL_MAX_LANE_WIDTH_DISABLE>"
  Lane Width Detection (LaneWDet)/1(LaneWDet_stLaneWDetFlg) -> Lane Condition Synthesis (LaneCSyn)/2(LaneCSyn_stLaneWDetFlg), Bus Creator/2  "LANE_WIDTH"
  Lane Condition Synthesis (LaneCSyn)/1(LaneCSyn_stLaneCSyn) -> LaneC_stLanCSyn/1  "LANE"
  Bus Selector/2 -> Lane Quality Disable Condition (LaneQlDC)/2(LaneQlDC_stFacmR0Ql)  "<R0_Q>"
  Bus Selector/1 -> Lane Quality Disable Condition (LaneQlDC)/1(LaneQlDC_stFacmL0Ql)  "<L0_Q>"
  LaneC_bsInInfoSyn/1 -> Bus Selector/1

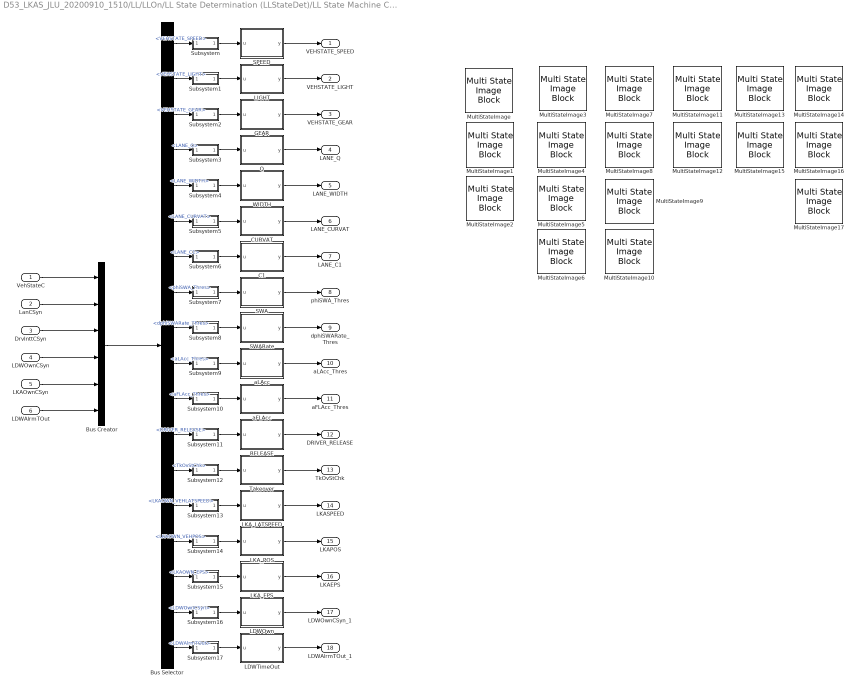
== system D53_LKAS_JLU_20200910_1510/LL/LLOn/LL State Determination (LLStateDet)/LL State Machine Conditions (LLSMCon)/Disable Condition (DisblC)/Subsystem ==
  VehStateC : Inport
  LanCSyn : Inport  Port=2
  DrvInttCSyn : Inport  Port=3
  LDWOwnCSyn : Inport  Port=4
  LKAOwnCSyn : Inport  Port=5
  LDWAlrmTOut : Inport  Port=6
  Bus Creator : BusCreator  Inputs=6
  Bus Selector : BusSelector  OutputSignals=VehStateC.VEHSTATE_SPEED,VehStateC.VEHSTATE_LIGHT,VehStateC.VEHSTATE_GEAR,LaneCSyn.LANE_Q,LaneCSyn.LANE_WIDTH,LaneCSyn.LANE_CURVAT,LaneCSyn.LANE_C1,DrvInttCSyn.DrvActnDet.phiSWA_Thres,DrvInttCSyn.DrvActnDet.dphiSWARate_Thres,DrvInttCSyn.DrvActnDet.aLAcc_Thres,DrvInttCSyn.DrvActnDet.aFLAcc_Thres,DrvInttCSyn.DRIVER_RELEASE,DrvInttCSyn.TkOvStChk,LKAOwnSyn.LKAOWN_VEHLATSPEED,LKAOwnSyn.LKAOWN_VEHPOS,LKAOwnSyn.LKAOWN_EPS,LDWOwnCSyn,LDWAlrmTOut
  C1 : MATLAB Function  TreatAsAtomicUnit=on
  CURVAT : MATLAB Function  TreatAsAtomicUnit=on
  GEAR : MATLAB Function  TreatAsAtomicUnit=on
  LDWOwn : MATLAB Function  TreatAsAtomicUnit=on
  LDWTimeOut : MATLAB Function  TreatAsAtomicUnit=on
  LIGHT : MATLAB Function  TreatAsAtomicUnit=on
  LKA_EPS : MATLAB Function  TreatAsAtomicUnit=on
  LKA_LATSPEED : MATLAB Function  TreatAsAtomicUnit=on
  LKA_POS : MATLAB Function  TreatAsAtomicUnit=on
  MultiStateImage : MultiStateImageBlock  WebBlockId=242577
  MultiStateImage1 : MultiStateImageBlock  WebBlockId=242578
  MultiStateImage10 : MultiStateImageBlock  WebBlockId=242579
  MultiStateImage11 : MultiStateImageBlock  WebBlockId=242580
  MultiStateImage12 : MultiStateImageBlock  WebBlockId=242581
  MultiStateImage13 : MultiStateImageBlock  WebBlockId=242582
  MultiStateImage14 : MultiStateImageBlock  WebBlockId=242583
  MultiStateImage15 : MultiStateImageBlock  WebBlockId=242584
  MultiStateImage16 : MultiStateImageBlock  WebBlockId=242585
  MultiStateImage17 : MultiStateImageBlock  WebBlockId=242586
  MultiStateImage2 : MultiStateImageBlock  WebBlockId=242587
  MultiStateImage3 : MultiStateImageBlock  WebBlockId=242588
  MultiStateImage4 : MultiStateImageBlock  WebBlockId=242589
  MultiStateImage5 : MultiStateImageBlock  WebBlockId=242590
  MultiStateImage6 : MultiStateImageBlock  WebBlockId=242591
  MultiStateImage7 : MultiStateImageBlock  WebBlockId=242592
  MultiStateImage8 : MultiStateImageBlock  WebBlockId=242593
  MultiStateImage9 : MultiStateImageBlock  WebBlockId=242594
  Q : MATLAB Function  TreatAsAtomicUnit=on
  RELEASE : MATLAB Function  TreatAsAtomicUnit=on
  SPEED : MATLAB Function  TreatAsAtomicUnit=on
  SWA : MATLAB Function  TreatAsAtomicUnit=on
  SWARate : MATLAB Function  TreatAsAtomicUnit=on
  Subsystem : Subsystem
  Subsystem1 : Subsystem
  Subsystem10 : Subsystem
  Subsystem11 : Subsystem
  Subsystem12 : Subsystem
  Subsystem13 : Subsystem
  Subsystem14 : Subsystem
  Subsystem15 : Subsystem
  Subsystem16 : Subsystem
  Subsystem17 : Subsystem
  Subsystem2 : Subsystem
  Subsystem3 : Subsystem
  Subsystem4 : Subsystem
  Subsystem5 : Subsystem
  Subsystem6 : Subsystem
  Subsystem7 : Subsystem
  Subsystem8 : Subsystem
  Subsystem9 : Subsystem
  Takeover : MATLAB Function  TreatAsAtomicUnit=on
  WIDTH : MATLAB Function  TreatAsAtomicUnit=on
  aFLAcc : MATLAB Function  TreatAsAtomicUnit=on
  aLAcc : MATLAB Function  TreatAsAtomicUnit=on
  VEHSTATE_SPEED : Outport
  VEHSTATE_LIGHT : Outport  Port=2
  VEHSTATE_GEAR : Outport  Port=3
  LANE_Q : Outport  Port=4
  LANE_WIDTH : Outport  Port=5
  LANE_CURVAT : Outport  Port=6
  LANE_C1 : Outport  Port=7
  phiSWA_Thres : Outport  Port=8
  dphiSWARate_Thres : Outport  Port=9
  aLAcc_Thres : Outport  Port=10
  aFLAcc_Thres : Outport  Port=11
  DRIVER_RELEASE : Outport  Port=12
  TkOvStChk : Outport  Port=13
  LKASPEED : Outport  Port=14
  LKAPOS : Outport  Port=15
  LKAEPS : Outport  Port=16
  LDWOwnCSyn_1 : Outport  Port=17
  LDWAlrmTOut_1 : Outport  Port=18
  wires:
  Bus Selector/16 -> Subsystem15/1(in1)  "<LKAOWN_EPS>"
  Subsystem15/1(Out1) -> LKA_EPS/1(u)
  LKA_EPS/1(y) -> LKAEPS/1
  Bus Selector/14 -> Subsystem13/1(in1)  "<LKAOWN_VEHLATSPEED>"
  Subsystem13/1(Out1) -> LKA_LATSPEED/1(u)
  LKA_LATSPEED/1(y) -> LKASPEED/1
  Subsystem17/1(Out1) -> LDWTimeOut/1(u)
  Subsystem14/1(Out1) -> LKA_POS/1(u)
  Subsystem16/1(Out1) -> LDWOwn/1(u)
  Subsystem11/1(Out1) -> RELEASE/1(u)
  Subsystem12/1(Out1) -> Takeover/1(u)
  Subsystem10/1(Out1) -> aFLAcc/1(u)
  Subsystem9/1(Out1) -> aLAcc/1(u)
  Subsystem8/1(Out1) -> SWARate/1(u)
  Subsystem7/1(Out1) -> SWA/1(u)
  Subsystem6/1(Out1) -> C1/1(u)
  Subsystem5/1(Out1) -> CURVAT/1(u)
  Subsystem4/1(Out1) -> WIDTH/1(u)
  Subsystem3/1(Out1) -> Q/1(u)
  Subsystem2/1(Out1) -> GEAR/1(u)
  Subsystem1/1(Out1) -> LIGHT/1(u)
  Subsystem/1(Out1) -> SPEED/1(u)
  Bus Selector/1 -> Subsystem/1(in1)  "<VEHSTATE_SPEED>"
  SPEED/1(y) -> VEHSTATE_SPEED/1
  LIGHT/1(y) -> VEHSTATE_LIGHT/1
  GEAR/1(y) -> VEHSTATE_GEAR/1
  aLAcc/1(y) -> aLAcc_Thres/1
  WIDTH/1(y) -> LANE_WIDTH/1
  LDWTimeOut/1(y) -> LDWAlrmTOut_1/1
  SWA/1(y) -> phiSWA_Thres/1
  aFLAcc/1(y) -> aFLAcc_Thres/1
  LDWAlrmTOut/1 -> Bus Creator/6
  Bus Selector/6 -> Subsystem5/1(in1)  "<LANE_CURVAT>"
  RELEASE/1(y) -> DRIVER_RELEASE/1
  SWARate/1(y) -> dphiSWARate_Thres/1
  Bus Selector/3 -> Subsystem2/1(in1)  "<VEHSTATE_GEAR>"
  LDWOwnCSyn/1 -> Bus Creator/4
  DrvInttCSyn/1 -> Bus Creator/3
  Bus Selector/5 -> Subsystem4/1(in1)  "<LANE_WIDTH>"
  C1/1(y) -> LANE_C1/1
  LanCSyn/1 -> Bus Creator/2
  Takeover/1(y) -> TkOvStChk/1
  Bus Selector/7 -> Subsystem6/1(in1)  "<LANE_C1>"
  Bus Selector/9 -> Subsystem8/1(in1)  "<dphiSWARate_Thres>"
  Bus Selector/2 -> Subsystem1/1(in1)  "<VEHSTATE_LIGHT>"
  Q/1(y) -> LANE_Q/1
  CURVAT/1(y) -> LANE_CURVAT/1
  Bus Selector/12 -> Subsystem11/1(in1)  "<DRIVER_RELEASE>"
  Bus Selector/10 -> Subsystem9/1(in1)  "<aLAcc_Thres>"
  Bus Selector/11 -> Subsystem10/1(in1)  "<aFLAcc_Thres>"
  Bus Selector/15 -> Subsystem14/1(in1)  "<LKAOWN_VEHPOS>"
  LDWOwn/1(y) -> LDWOwnCSyn_1/1
  LKA_POS/1(y) -> LKAPOS/1
  Bus Selector/18 -> Subsystem17/1(in1)  "<LDWAlrmTOut>"
  Bus Selector/4 -> Subsystem3/1(in1)  "<LANE_Q>"
  VehStateC/1 -> Bus Creator/1
  Bus Creator/1 -> Bus Selector/1
  Bus Selector/17 -> Subsystem16/1(in1)  "<LDWOwnCSyn>"
  LKAOwnCSyn/1 -> Bus Creator/5
  Bus Selector/8 -> Subsystem7/1(in1)  "<phiSWA_Thres>"
  Bus Selector/13 -> Subsystem12/1(in1)  "<TkOvStChk>"

== system D53_LKAS_JLU_20200910_1510/LL/LLOn/LL State Determination (LLStateDet)/LL State Machine Conditions (LLSMCon)/Disable Condition (DisblC)/Vehicle State Condition (VehStateC) ==
  VehStateC_stDACMode : Inport
  VehStateC_bsInInfoSyn : Inport  Port=2
  VehStateC_bsLLSMConClb : Inport  Port=3
  Bus Creator : BusCreator  Inputs=3
  Bus Selector : BusSelector  OutputSignals=bsVehMovInfo.ESC_VehSpd,bsBCMInfo,bsPTState.TCU_ActualGear
  Bus Selector1 : BusSelector  OutputSignals=DisblCClb.LL_MAX_LDWS_SPEED_DISABLE,DisblCClb.LL_MAX_LKAS_SPEED_DISABLE,DisblCClb.LL_MIN_LKAS_SPEED_DISABLE
  Emergency Light Enable Condition (EmgcyLghtEC) : Subsystem  Description=|
      | Block Name: Emergency Light Enable Condition
      | Ab.: EmgcyLghtEC
      | No.: 1.1.1.2.1.3
      | Rev: 0.0.1
      | Update Date: 19-3-26
  Gear Disable Condition (GearDC) : Subsystem  Description=|
      | Block Name: Gear Disable Condition
      | Ab.: GearDC
      | No.: 1.1.1.3.1.4
      | Rev: 0.0.1
      | Update Date: 19-3-26
  Vehicle Speed Disable Condition (VehSpdDC) : Subsystem  Description=|
      | Block Name: Vehicle Speed Disable Condition
      | Ab.: VehSpdDC
      | No.: 1.1.1.3.1.1
      | Rev: 0.0.1
      | Update Date: 19-3-26
  Vehicle State Condition Synthesis (VehStateCSyn) : Subsystem  Description=|
      | Block Name: Vehicle State Condition Synthesis
      | Ab.: VehStateCSyn
      | No.: 1.1.1.3.1.5
      | Rev: 0.0.1
      | Update Date: 19-3-26
  VehStateC_stVehStateCSyn : Outport
  VehStateC : Outport  Port=2
  wires:
  Bus Creator/1 -> VehStateC/1  "VehStateC"
  Bus Selector/2 -> Emergency Light Enable Condition (EmgcyLghtEC)/1(EmgcyLghtEC_bsStLampState)  "<bsBCMInfo>"
  Gear Disable Condition (GearDC)/1(GearDC_stGearDCFlg) -> Bus Creator/3, Vehicle State Condition Synthesis (VehStateCSyn)/3(VehStateCSyn_stGearDCFlg)  "VEHSTATE_GEAR"
  Bus Selector/3 -> Gear Disable Condition (GearDC)/1(In1)  "<TCU_ActualGear>"
  Emergency Light Enable Condition (EmgcyLghtEC)/1(EmgcyLghtEC_stEmgcyLghtECFlg) -> Vehicle State Condition Synthesis (VehStateCSyn)/2(VehStateCSyn_stEmgcyLghtDCFlg), Bus Creator/2  "VEHSTATE_LIGHT"
  Bus Selector1/2 -> Vehicle Speed Disable Condition (VehSpdDC)/4(VehSpdDC_vLKAVehSpdMax_C)  "<LL_MAX_LKAS_SPEED_DISABLE>"
  Bus Selector1/3 -> Vehicle Speed Disable Condition (VehSpdDC)/5(VehSpdDC_vVehSpdMin_C)  "<LL_MIN_LKAS_SPEED_DISABLE>"
  VehStateC_bsLLSMConClb/1 -> Bus Selector1/1
  VehStateC_stDACMode/1 -> Vehicle Speed Disable Condition (VehSpdDC)/1(VehSpdDC_stDACMode)
  Bus Selector1/1 -> Vehicle Speed Disable Condition (VehSpdDC)/3(VehSpdDC_vLDWVehSpdMax_C)  "<LL_MAX_LDWS_SPEED_DISABLE>"
  Vehicle Speed Disable Condition (VehSpdDC)/1(VehSpdDC_stVehSpdDCFlg) -> Vehicle State Condition Synthesis (VehStateCSyn)/1(VehStateCSyn_stVehSpdDCFlg), Bus Creator/1  "VEHSTATE_SPEED"
  Bus Selector/1 -> Vehicle Speed Disable Condition (VehSpdDC)/2(VehSpdDC_vVehSpd)  "<ESC_VehSpd>"
  Vehicle State Condition Synthesis (VehStateCSyn)/1(VehStateCSyn_stVehStateCSyn) -> VehStateC_stVehStateCSyn/1  "VEHSTATE"
  VehStateC_bsInInfoSyn/1 -> Bus Selector/1

== system D53_LKAS_JLU_20200910_1510/LL/LLOn/LL State Determination (LLStateDet)/LL State Machine Conditions (LLSMCon)/Enable Condition (EnaC)/Driver Intent Condition (DrvInttC) ==
  DrvInttC_bsInInfoSyn : Inport
  DrvInttC_bsLLSMConClb : Inport  Port=2
  Abs{1..4} (4 alike) : Abs  OutDataTypeStr=single
  Bus Selector : BusSelector  OutputSignals=bsSWAInfo.SW_Angle,bsEPSInfo.EPS_SW_Trq,bsVehMovInfo.ESC_LatAcc,bsVehMovInfo.ESC_LonAcc
  Bus Selector1 : BusSelector  OutputSignals=EnaCClb.LL_MAX_STEER_ANGLE_ENABLE,EnaCClb.LL_MAX_STEER_SPEED_ENABLE,EnaCClb.LL_MAX_DRIVER_TORQUE_ENABLE,EnaCClb.LL_MAX_LAT_ACC_ENABLE,EnaCClb.LL_MAX_LONG_ACC_ENABLE,EnaCClb.LL_MAX_LONG_DECEL_ENABLE
  Discrete Derivative : simulink/Discrete/Discrete Derivative  gainval=1.0  ICPrevScaledInput=0.0  OutMin=[]  OutMax=[]  OutDataTypeStr=single  OutputDataTypeScalingMode=single  OutDataType=fixdt(1, 16)  OutScaling=2^-10  DoSatur=off
  Interval Test Dynamic : simulink/Logic and Bit Operations/Interval Test Dynamic  IntervalClosedRight=off  IntervalClosedLeft=off  OutDataTypeStr=boolean
      settings: SourceProductName=Simulink  SourceProductBaseCode=SL
  Logical Operator3 : Logic  Inputs=5  AllPortsSameDT=off  OutDataTypeStr=boolean
  Relational Operator{,1..3} (4 alike) : RelationalOperator  Operator=<  OutDataTypeStr=boolean  RndMeth=Nearest
  Unary Minus : UnaryMinus
  DrvInttC_stDrvInttCSyn : Outport
  wires:
  Relational Operator/1 -> Logical Operator3/3
  Relational Operator1/1 -> Logical Operator3/1
  Abs2/1 -> Relational Operator1/1
  Abs3/1 -> Relational Operator2/1
  Discrete Derivative/1 -> Abs3/1
  Relational Operator2/1 -> Logical Operator3/2
  Abs4/1 -> Relational Operator3/1
  Abs1/1 -> Relational Operator/1
  Unary Minus/1 -> Interval Test Dynamic/3
  Relational Operator3/1 -> Logical Operator3/4
  Interval Test Dynamic/1 -> Logical Operator3/5
  Logical Operator3/1 -> DrvInttC_stDrvInttCSyn/1  "DRIVERINT_ACTION"
  DrvInttC_bsLLSMConClb/1 -> Bus Selector1/1
  Bus Selector1/6 -> Unary Minus/1  "<LL_MAX_LONG_DECEL_ENABLE>"
  Bus Selector1/5 -> Interval Test Dynamic/1  "<LL_MAX_LONG_ACC_ENABLE>"
  Bus Selector1/4 -> Relational Operator3/2  "<LL_MAX_LAT_ACC_ENABLE>"
  Bus Selector1/3 -> Relational Operator/2  "<LL_MAX_DRIVER_TORQUE_ENABLE>"
  Bus Selector1/2 -> Relational Operator2/2  "<LL_MAX_STEER_SPEED_ENABLE>"
  Bus Selector1/1 -> Relational Operator1/2  "<LL_MAX_STEER_ANGLE_ENABLE>"
  Bus Selector/4 -> Interval Test Dynamic/2  "<ESC_LonAcc>"
  Bus Selector/3 -> Abs4/1  "<ESC_LatAcc>"
  Bus Selector/1 -> Discrete Derivative/1, Abs2/1  "<SW_Angle>"
  Bus Selector/2 -> Abs1/1  "<EPS_SW_Trq>"
  DrvInttC_bsInInfoSyn/1 -> Bus Selector/1

== system D53_LKAS_JLU_20200910_1510/LL/LLOn/LL State Determination (LLStateDet)/LL State Machine Conditions (LLSMCon)/Enable Condition (EnaC)/Enable Condition Synthesis (EnaCSyn) ==
  EnaCSyn_stDACMode : Inport
  EnaCSyn_stVehStateC : Inport  Port=2
  EnaCSyn_stLaneC : Inport  Port=3
  EnaCSyn_stDrvInttC : Inport  Port=4
  EnaCSyn_stLDWOwnC : Inport  Port=5
  EnaCSyn_stLKAOwnC : Inport  Port=6
  Cast To Single : DataTypeConversion  OutDataTypeStr=uint8
  Cast To Single1 : DataTypeConversion  OutDataTypeStr=uint8
  Cast To Single2 : DataTypeConversion  OutDataTypeStr=uint8
  If : If  NumInputs=2  IfExpression=(u1 ==1|u1==2)& u2 == 1
  If Action Subsystem : Subsystem  TreatAsAtomicUnit=on
  If Action Subsystem2 : Subsystem  TreatAsAtomicUnit=on
  If Action Subsystem3 : Subsystem  TreatAsAtomicUnit=on
  If Action Subsystem4 : Subsystem  TreatAsAtomicUnit=on
  If1 : If  NumInputs=2  IfExpression=u1 == 2 & u2 == 1
  Logical Operator1 : Logic  AllPortsSameDT=off  OutDataTypeStr=boolean
  Logical Operator2 : Logic  Inputs=3  AllPortsSameDT=off  OutDataTypeStr=boolean
  Logical Operator3 : Logic  AllPortsSameDT=off  OutDataTypeStr=boolean
  Merge : Merge
  Merge1 : Merge
  EnaCSyn_stLDWEnaCSyn : Outport
  EnaCSyn_stLKAEnaCSyn : Outport  Port=2
  wires:
  Cast To Single2/1 -> If1/2
  Cast To Single1/1 -> If/2
  Cast To Single/1 -> If/1, If1/1
  Logical Operator1/1 -> Cast To Single2/1
  If Action Subsystem4/1(Out) -> Merge1/2
  Merge1/1 -> EnaCSyn_stLKAEnaCSyn/1
  If1/2 -> If Action Subsystem4/Action
  If1/1 -> If Action Subsystem2/Action
  If Action Subsystem2/1(Out) -> Merge1/1
  If Action Subsystem3/1(Out) -> Merge/2
  EnaCSyn_stLKAOwnC/1 -> Logical Operator1/2
  Logical Operator2/1 -> Logical Operator3/2, Logical Operator1/1
  EnaCSyn_stDACMode/1 -> Cast To Single/1
  Merge/1 -> EnaCSyn_stLDWEnaCSyn/1
  Logical Operator3/1 -> Cast To Single1/1
  EnaCSyn_stLDWOwnC/1 -> Logical Operator3/1
  If/2 -> If Action Subsystem3/Action
  If/1 -> If Action Subsystem/Action
  If Action Subsystem/1(Out) -> Merge/1
  EnaCSyn_stDrvInttC/1 -> Logical Operator2/3
  EnaCSyn_stLaneC/1 -> Logical Operator2/2
  EnaCSyn_stVehStateC/1 -> Logical Operator2/1

== system D53_LKAS_JLU_20200910_1510/LL/LLOn/LL State Determination (LLStateDet)/LL State Machine Conditions (LLSMCon)/Enable Condition (EnaC)/LDW Own Condition (LDWOwnC) ==
  LDWOwnC_stDACMode : Inport
  LDWOwnC_LaneWidth : Inport  Port=2
  LDWOwnC_bsPrDvtInfo : Inport  Port=3
  LDWOwnC_bsLLSMConClb : Inport  Port=4
  Bus Selector1 : BusSelector  OutputSignals=EnaCClb.LL_LDW_EarliestWarnLine_C
  LDW Own Condition Synthesis (LDWOwnCSyn) : Subsystem  Description=|
      | Block Name: LDW Own Condition Synthesis
      | Ab.: LDWOwnCSyn
      | No.: 1.1.1.2.4.2
      | Rev: 0.0.1
      | Update Date: 19-3-26
  Vehicle Position Check (VehPosChk) : Subsystem  Description=|
      | Block Name: Vehicle Position Check
      | Ab.: VehPosChk
      | No.: 1.1.1.2.4.1
      | Rev: 0.0.1
      | Update Date: 19-3-26
  LDWOwnC_stLDWOwnCSyn : Outport
  wires:
  LDWOwnC_LaneWidth/1 -> Vehicle Position Check (VehPosChk)/1(VehPosChk_LaneWidth)
  LDWOwnC_bsPrDvtInfo/1 -> Vehicle Position Check (VehPosChk)/2(VehPosChk_bsDvtInfo)
  Bus Selector1/1 -> Vehicle Position Check (VehPosChk)/3(VehPosChk_lWarnLine_C)  "<LL_LDW_EarliestWarnLine_C>"
  LDWOwnC_bsLLSMConClb/1 -> Bus Selector1/1
  LDWOwnC_stDACMode/1 -> LDW Own Condition Synthesis (LDWOwnCSyn)/1(LDWOwnCSyn_stDACMode)
  Vehicle Position Check (VehPosChk)/1(VehPosChk_stVehPosChk) -> LDW Own Condition Synthesis (LDWOwnCSyn)/2(LDWOwnCSyn_stVehPosChk)
  LDW Own Condition Synthesis (LDWOwnCSyn)/1(LDWOwnCSyn_stLDWOwnCSyn) -> LDWOwnC_stLDWOwnCSyn/1
